simulink model "enumdef_mcos4"  (R2022b)
settings: Solver=VariableStepAuto  StartTime=0.0  StopTime=10.0  RelTol=1e-3
model workspace (MAT data in the model file):
  var_green : enumdef_rgb (value not decoded)
  var_red : enumdef_rgb (value not decoded)
  var_yes : enumdef_yesno (value not decoded)
symbols that are objects in the model workspace (value not decoded): var_green, var_red, var_yes
settings Model: Creator=ntwigg  LastModifiedBy=ntwigg

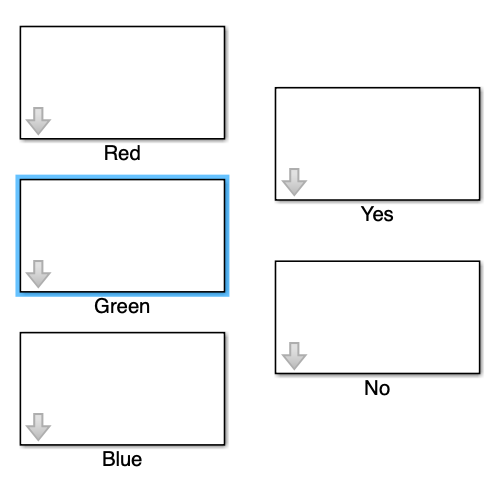
[thumbnail: Simulink's stored preview of the top-level diagram]
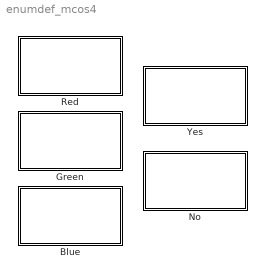
== system enumdef_mcos4 ==
  Blue : Subsystem  mask{Color=blue (3)}
  Green : Subsystem  mask{Color=var_green}
  No : Subsystem  mask{YesNo=no (2)}
  Red : Subsystem  mask{Color=var_red}
  Yes : Subsystem  mask{YesNo=var_yes}

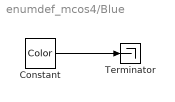
== system enumdef_mcos4/Blue ==
  Constant : Constant  Value=Color
  Terminator : Terminator
  wires:
  Constant/1 -> Terminator/1

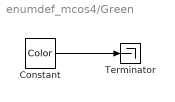
== system enumdef_mcos4/Green ==
  Constant : Constant  Value=Color
  Terminator : Terminator
  wires:
  Constant/1 -> Terminator/1

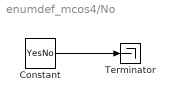
== system enumdef_mcos4/No ==
  Constant : Constant  Value=YesNo
  Terminator : Terminator
  wires:
  Constant/1 -> Terminator/1

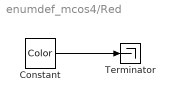
== system enumdef_mcos4/Red ==
  Constant : Constant  Value=Color
  Terminator : Terminator
  wires:
  Constant/1 -> Terminator/1

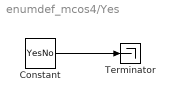
== system enumdef_mcos4/Yes ==
  Constant : Constant  Value=YesNo
  Terminator : Terminator
  wires:
  Constant/1 -> Terminator/1
